simulink model "model_v3"  (R2019a)
settings: Solver=VariableStepAuto  StartTime=0.0  StopTime=12.0  RelTol=1e-3
values from neighbouring files (symbols this model uses):
  m = 200    [config_v3.m]
libraries: simulink x4, simulink_extras x3
settings Model: Creator=jacoboffersen  LastModifiedBy=jacoboffersen

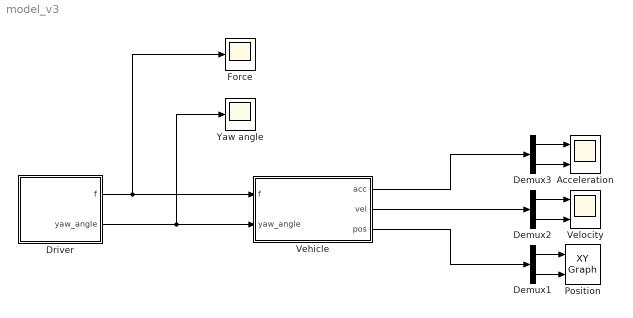
== system model_v3 ==
  Acceleration : Scope  NumInputPorts=2
  Demux1 : Demux  Outputs=2
  Demux2 : Demux  Outputs=2
  Demux3 : Demux  Outputs=2
  Driver : Subsystem
  Force : Scope
  Position : simulink/Sinks/XY Graph  xmin=-1  xmax=1  ymin=-1  ymax=1  st=-1
  Vehicle : Subsystem
  Velocity : Scope  NumInputPorts=2
  Yaw angle : Scope
  wires:
  Driver/1(f) -> Force/1, Vehicle/1(f)
  Demux1/2 -> Position/2
  Demux1/1 -> Position/1
  Vehicle/1(acc) -> Demux3/1
  Vehicle/2(vel) -> Demux2/1
  Vehicle/3(pos) -> Demux1/1
  Driver/2(yaw_angle) -> Yaw angle/1, Vehicle/2(yaw_angle)
  Demux2/1 -> Velocity/1
  Demux2/2 -> Velocity/2
  Demux3/1 -> Acceleration/1
  Demux3/2 -> Acceleration/2

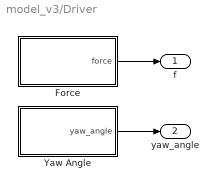
== system model_v3/Driver ==
  Force : Subsystem
  Yaw Angle : Subsystem
  f : Outport
  yaw_angle : Outport  Port=2
  wires:
  Yaw Angle/1(yaw_angle) -> yaw_angle/1
  Force/1(force) -> f/1

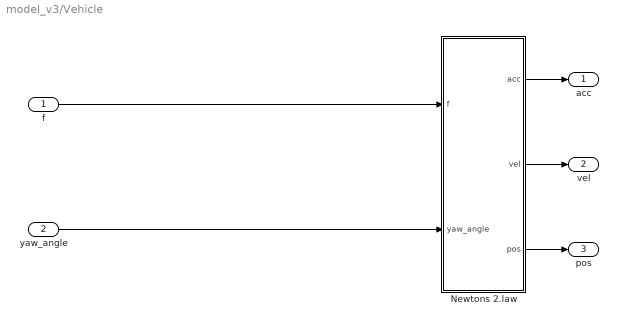
== system model_v3/Vehicle ==
  f : Inport
  yaw_angle : Inport  Port=2
  Newtons 2.law : Subsystem
  acc : Outport
  vel : Outport  Port=2
  pos : Outport  Port=3
  wires:
  Newtons 2.law/1(acc) -> acc/1
  Newtons 2.law/2(vel) -> vel/1
  Newtons 2.law/3(pos) -> pos/1
  yaw_angle/1 -> Newtons 2.law/2(yaw_angle)
  f/1 -> Newtons 2.law/1(f)

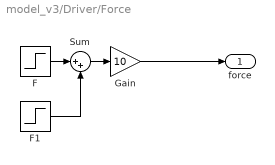
== system model_v3/Driver/Force ==
  F : Step  SampleTime=0
  F1 : Step  Time=3  After=-1  SampleTime=0
  Gain : Gain  Gain=10
  Sum : Sum  Inputs=|++
  force : Outport
  wires:
  F1/1 -> Sum/2
  F/1 -> Sum/1
  Sum/1 -> Gain/1
  Gain/1 -> force/1

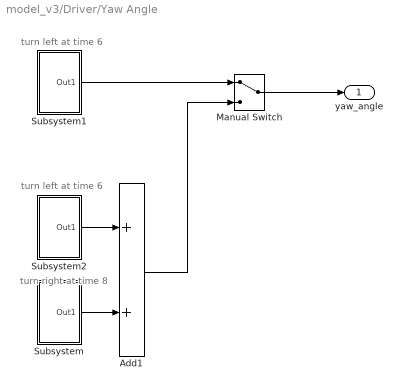
== system model_v3/Driver/Yaw Angle ==
  note: turn right at time 8
  note: turn left at time 6
  note: turn left at time 6
  Add1 : Sum
  Manual Switch : ManualSwitch
  Subsystem : Subsystem
  Subsystem1 : Subsystem
  Subsystem2 : Subsystem
  yaw_angle : Outport
  wires:
  Add1/1 -> Manual Switch/2
  Manual Switch/1 -> yaw_angle/1
  Subsystem/1(Out1) -> Add1/2
  Subsystem1/1(Out1) -> Manual Switch/1
  Subsystem2/1(Out1) -> Add1/1

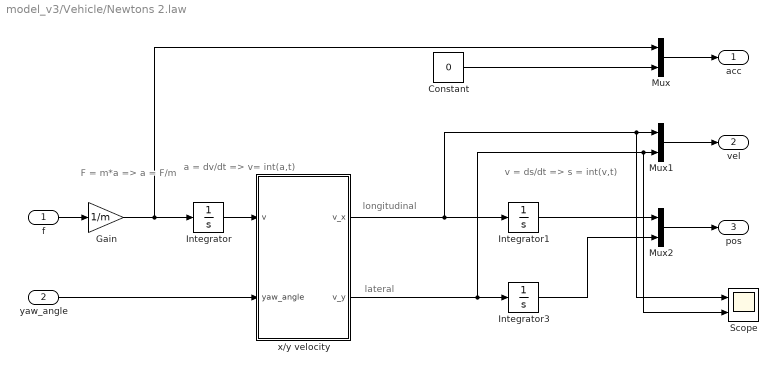
== system model_v3/Vehicle/Newtons 2.law ==
  note: lateral
  note: longitudinal
  note: a = dv/dt =>
      | v= int(a,t)
  note: v = ds/dt =>
      | s = int(v,t)
  note: F = m*a =>
      | a = F/m
  f : Inport
  yaw_angle : Inport  Port=2
  Constant : Constant  Value=0
  Gain : Gain  Gain=1/m
  Integrator : Integrator
  Integrator1 : Integrator
  Integrator3 : Integrator
  Mux : Mux  Inputs=2
  Mux1 : Mux  Inputs=2
  Mux2 : Mux  Inputs=2
  Scope : Scope  NumInputPorts=2
  x/y velocity : Subsystem
  acc : Outport
  vel : Outport  Port=2
  pos : Outport  Port=3
  wires:
  Gain/1 -> Mux/1, Integrator/1
  Mux1/1 -> vel/1
  Mux/1 -> acc/1
  Mux2/1 -> pos/1
  Integrator3/1 -> Mux2/2
  Integrator1/1 -> Mux2/1
  f/1 -> Gain/1
  Constant/1 -> Mux/2
  x/y velocity/1(v_x) -> Scope/1, Mux1/1, Integrator1/1
  x/y velocity/2(v_y) -> Scope/2, Mux1/2, Integrator3/1
  Integrator/1 -> x/y velocity/1(v)
  yaw_angle/1 -> x/y velocity/2(yaw_angle)

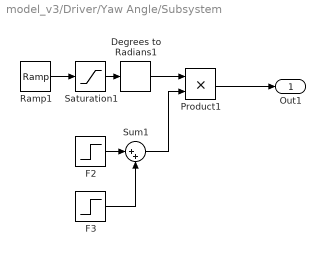
== system model_v3/Driver/Yaw Angle/Subsystem ==
  Degrees to Radians1 : simulink_extras/Transformations/Degrees to Radians
  F2 : Step  Time=8  SampleTime=0
  F3 : Step  Time=12  After=-1  SampleTime=0
  Product1 : Product
  Ramp1 : simulink/Sources/Ramp  slope=-15  start=8  InitialOutput=30
  Saturation1 : Saturate  UpperLimit=30  LowerLimit=-30
  Sum1 : Sum  Inputs=|++
  Out1 : Outport
  wires:
  Degrees to Radians1/1 -> Product1/1
  Saturation1/1 -> Degrees to Radians1/1
  F2/1 -> Sum1/1
  Product1/1 -> Out1/1
  F3/1 -> Sum1/2
  Sum1/1 -> Product1/2
  Ramp1/1 -> Saturation1/1

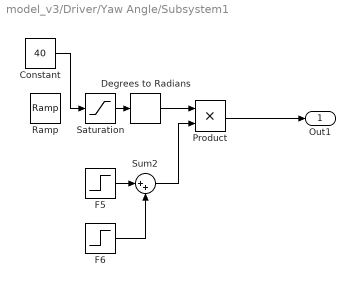
== system model_v3/Driver/Yaw Angle/Subsystem1 ==
  Constant : Constant  Value=40
  Degrees to Radians : simulink_extras/Transformations/Degrees to Radians
  F5 : Step  Time=6  SampleTime=0
  F6 : Step  Time=8  After=-1  SampleTime=0
  Product : Product
  Ramp : simulink/Sources/Ramp  slope=15  start=6  InitialOutput=0
  Saturation : Saturate  UpperLimit=30  LowerLimit=-30
  Sum2 : Sum  Inputs=|++
  Out1 : Outport
  wires:
  Degrees to Radians/1 -> Product/1
  F6/1 -> Sum2/2
  Sum2/1 -> Product/2
  Product/1 -> Out1/1
  Saturation/1 -> Degrees to Radians/1
  F5/1 -> Sum2/1
  Constant/1 -> Saturation/1

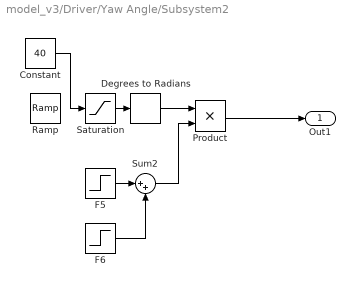
== system model_v3/Driver/Yaw Angle/Subsystem2 ==
  Constant : Constant  Value=40
  Degrees to Radians : simulink_extras/Transformations/Degrees to Radians
  F5 : Step  Time=6  SampleTime=0
  F6 : Step  Time=8  After=-1  SampleTime=0
  Product : Product
  Ramp : simulink/Sources/Ramp  slope=15  start=6  InitialOutput=0
  Saturation : Saturate  UpperLimit=30  LowerLimit=-30
  Sum2 : Sum  Inputs=|++
  Out1 : Outport
  wires:
  Degrees to Radians/1 -> Product/1
  F6/1 -> Sum2/2
  Sum2/1 -> Product/2
  Product/1 -> Out1/1
  Saturation/1 -> Degrees to Radians/1
  F5/1 -> Sum2/1
  Constant/1 -> Saturation/1

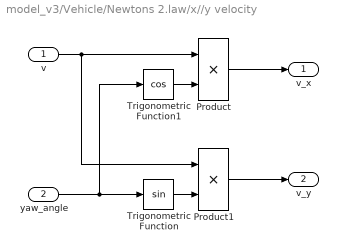
== system model_v3/Vehicle/Newtons 2.law/x//y velocity ==
  v : Inport
  yaw_angle : Inport  Port=2
  Product : Product
  Product1 : Product
  Trigonometric Function : Trigonometry
  Trigonometric Function1 : Trigonometry  Operator=cos
  v_x : Outport
  v_y : Outport  Port=2
  wires:
  Product1/1 -> v_y/1
  v/1 -> Product1/1, Product/1
  yaw_angle/1 -> Trigonometric Function1/1, Trigonometric Function/1
  Trigonometric Function1/1 -> Product/2
  Product/1 -> v_x/1
  Trigonometric Function/1 -> Product1/2
